simulink model "TrafficLight"  (R2021b)
settings: Solver=FixedStepDiscrete  StartTime=0.0  StopTime=10.0  RelTol=1e-3  EnableMultiTasking=on
settings Model: Creator=fady  LastModifiedBy=fady
settings DataIOCC: ReturnWorkspaceOutputs=off
settings OptimizationCC: DefaultParameterBehavior=Inlined  InlineInvariantSignals=on  EnableMemcpy=off  LifeSpan=1  EfficientTunableParamExpr=on
settings DebuggingCC: UnderspecifiedInitializationDetection=Classic  MergeDetectMultiDrivingBlocksExec=none  SFMachineParentedDataDiag=warning  ArithmeticOperatorsInVariantConditions=warning
settings ModelReferenceCC: PropagateSignalLabelsOutOfModel=off
settings SFSimCC: MATLABDynamicMemAlloc=off  CustomCodeUndefinedFunction=UseInterfaceOnly
settings RTWCC: Description=Embedded Coder  SystemTargetFile=ert.tlc  GenCodeOnly=on  TemplateMakefile=ert_default_tmf  GenerateReport=on  IncludeHyperlinkInReport=on  LaunchReport=on  GenerateTraceInfo=on  GenerateTraceReport=on  GenerateTraceReportSl=on  GenerateTraceReportSf=on  GenerateTraceReportEml=on
settings CodeAppCC: ForceParamTrailComments=on  IgnoreCustomStorageClasses=off  OperatorAnnotations=on  SimulinkDataObjDesc=on  SFDataObjDesc=on  MATLABFcnDesc=on  InsertBlockDesc=on  StateflowObjectComments=on  MATLABSourceComments=on
settings ERTTargetCC: MultiwordLength=2048  GenerateSampleERTMain=on  InlinedParameterPlacement=NonHierarchical  ERTCustomFileTemplate=example_file_process.tlc

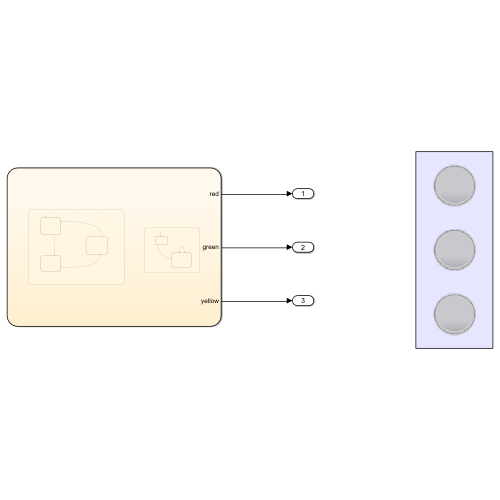
[thumbnail: Simulink's stored preview of the top-level diagram]
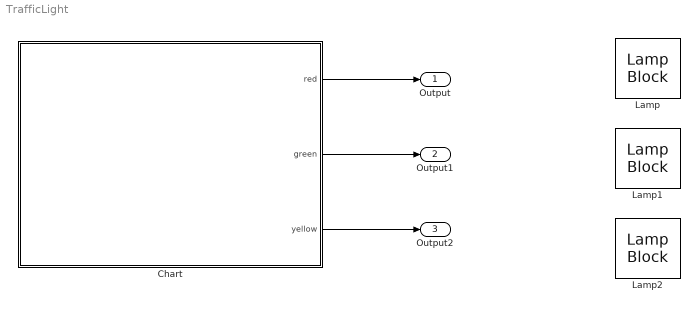
== system TrafficLight ==
  Chart : Stateflow chart  TreatAsAtomicUnit=on
  Lamp : LampBlock  LabelPosition=Hide
  Lamp1 : LampBlock  LabelPosition=Hide
  Lamp2 : LampBlock  LabelPosition=Hide
  Output : Outport
  Output1 : Outport  Port=2
  Output2 : Outport  Port=3
  wires:
  Chart/1(red) -> Output/1
  Chart/2(green) -> Output1/1
  Chart/3(yellow) -> Output2/1

== stateflow chart TrafficLight/Chart ==
  state TrafficLight [parallel]
    en:
    red = 0;
    yellow = 0;
    green = 0;
    count = 0;
    settings: executionOrder=1
    state Red
      du:
      red = 1;
      ex:
      red = 0;
    state Yellow
      du:
      yellow = 1;
      ex:
      yellow = 0;
    state Green
      du:
      green = 1;
      ex:
      green = 0
    (default) -> Red
    Yellow -> Red : [count == 1]
    Red -> Green : [count == 1]
    Green -> Yellow : [count == 1]
  state Counter [parallel]
    settings: executionOrder=2
    state init
      en:
      count = 0;
    state Count
      en:
      count = 1;
      du:
      count = 0;
    (default) -> init
    init -> Count : after(3,tick)
    Count -> Count : after(3, tick)
  data: count local double =0; red output double =0; green output double =0; yellow output double =0
